simulink model "model"  (R2015a)
settings: Solver=ode45  StartTime=0.0  StopTime=20  RelTol=1e-3
values from neighbouring files (symbols this model uses):
  J = 0.003    [model_sim.m]
  ke = 0.53    [model_sim.m]
  kE = 46.6    [model_sim.m]
  kf = 0.0005    [model_sim.m]
  km = 0.53    [model_sim.m]
  kMi = 1.63    [model_sim.m]
  kMw = 0.023    [model_sim.m]
  Ra = 2    [model_sim.m]
  Ta = 0.11    [model_sim.m]
  Tu = 0.002    [model_sim.m]
settings Model: Creator=B014-5  LastModifiedBy=B014-5

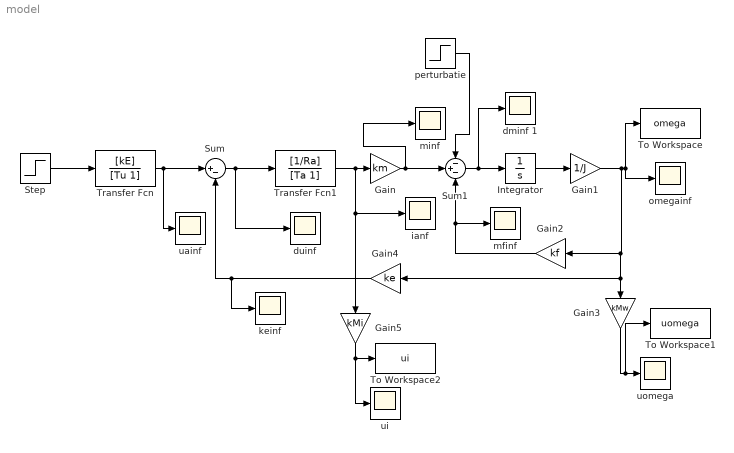
== system model ==
  Gain : Gain  Gain=km
  Gain1 : Gain  Gain=1/J
  Gain2 : Gain  Gain=kf
  Gain3 : Gain  Gain=kMw
  Gain4 : Gain  Gain=ke
  Gain5 : Gain  Gain=kMi
  Integrator : Integrator
  Step : Step  Time=0  After=3  SampleTime=0
  Sum : Sum  Inputs=|+-
  Sum1 : Sum  Inputs=-+-
  To Workspace : ToWorkspace  VariableName=omega  SampleTime=-1
      settings: Save2DSignal=2-D array (concatenate along first dimension)
  To Workspace1 : ToWorkspace  VariableName=uomega  SampleTime=-1
      settings: Save2DSignal=2-D array (concatenate along first dimension)
  To Workspace2 : ToWorkspace  VariableName=ui  SampleTime=-1
      settings: Save2DSignal=2-D array (concatenate along first dimension)
  Transfer Fcn : TransferFcn  Numerator=[kE]  Denominator=[Tu 1]
  Transfer Fcn1 : TransferFcn  Numerator=[1/Ra]  Denominator=[Ta 1]
  dminf 1 : Scope
      settings: SaveName=ScopeData8
  "duinf " : Scope
      settings: SaveName=ScopeData4
  ianf : Scope
      settings: SaveName=ScopeData5
  "keinf " : Scope
      settings: SaveName=ScopeData9
  mfinf : Scope
      settings: SaveName=ScopeData7
  minf : Scope
      settings: SaveName=ScopeData6
  omegainf : Scope
  perturbatie : Step  Time=10  After=0  SampleTime=0
  uainf : Scope
      settings: SaveName=ScopeData3
  ui : Scope
      settings: SaveName=ScopeData2
  "uomega " : Scope
  wires:
  Transfer Fcn/1 -> uainf/1, Sum/1
  Sum/1 -> "duinf "/1, Transfer Fcn1/1
  Transfer Fcn1/1 -> Gain5/1, ianf/1, Gain/1
  Sum1/1 -> dminf 1/1, Integrator/1
  Integrator/1 -> Gain1/1
  Gain1/1 -> Gain4/1, Gain3/1, Gain2/1, To Workspace/1, omegainf/1
  Gain3/1 -> To Workspace1/1, "uomega "/1
  Gain2/1 -> Sum1/3, mfinf/1
  Gain4/1 -> "keinf "/1, Sum/2
  Gain5/1 -> ui/1, To Workspace2/1
  Step/1 -> Transfer Fcn/1
  perturbatie/1 -> Sum1/1
  Gain/1 -> minf/1, Sum1/2
